simulink model "Stand_Balance"  (R2021b)
settings: Solver=FixedStepDiscrete  StartTime=0.0  StopTime=inf  FixedStep=0.0005  RelTol=1e-3
libraries: simulink x4, IFR_StackLiteDualDrive_SimulinkLib x4
settings Model: Creator=ysl  LastModifiedBy=ysl
settings OptimizationCC: DefaultParameterBehavior=Inlined  EnhancedBackFolding=on  PassReuseOutputArgsAs=Individual arguments  ZeroExternalMemoryAtStartup=off  ZeroInternalMemoryAtStartup=off  OptimizeBlockOrder=speed  DifferentSizesBufferReuse=on  OptimizationCustomize=off  EfficientTunableParamExpr=on
settings DebuggingCC: ParameterTunabilityLossMsg=error
settings SFSimCC: MATLABDynamicMemAlloc=off
settings RTWCC: Description=IFR StackLite-DualDrive Base on stm32f405RGT6  SystemTargetFile=stacklite_dualdrive.tlc  TemplateMakefile=stacklite_dualdrive.tmf  GenerateReport=on
settings CodeAppCC: ForceParamTrailComments=on  IgnoreCustomStorageClasses=off  OperatorAnnotations=on  SimulinkDataObjDesc=on  SFDataObjDesc=on  InsertBlockDesc=on
settings STFCustomTargetCC: TargetLangStandard=C99 (ISO)  MultiwordLength=256  ParMdlRefBuildCompliant=on  CompOptLevelCompliant=on  CombineOutputUpdateFcns=on  ERTCustomFileBanners=on  SupportContinuousTime=off  SupportNonInlinedSFcns=off  RemoveResetFunc=on  MATLABClassNameForMDSCustomization=Simulink.SoftwareTarget.ERTCustomization  CPPClassGenCompliant=on  GRTInterface=off  SystemTargetFile=stacklite_dualdrive.tlc
settings ERTTargetCC: TargetLangStandard=C99 (ISO)  ConcurrentExecutionCompliant=off  ModelStepFunctionPrototypeControlCompliant=off  UseToolchainInfoCompliant=off  InlinedParameterPlacement=NonHierarchical  ERTCustomFileTemplate=example_file_process.tlc

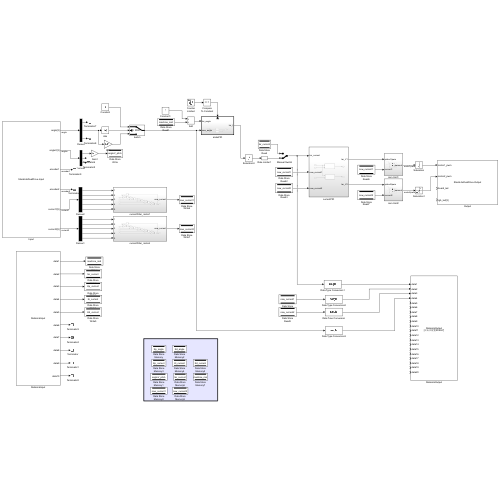
[thumbnail: Simulink's stored preview of the top-level diagram]
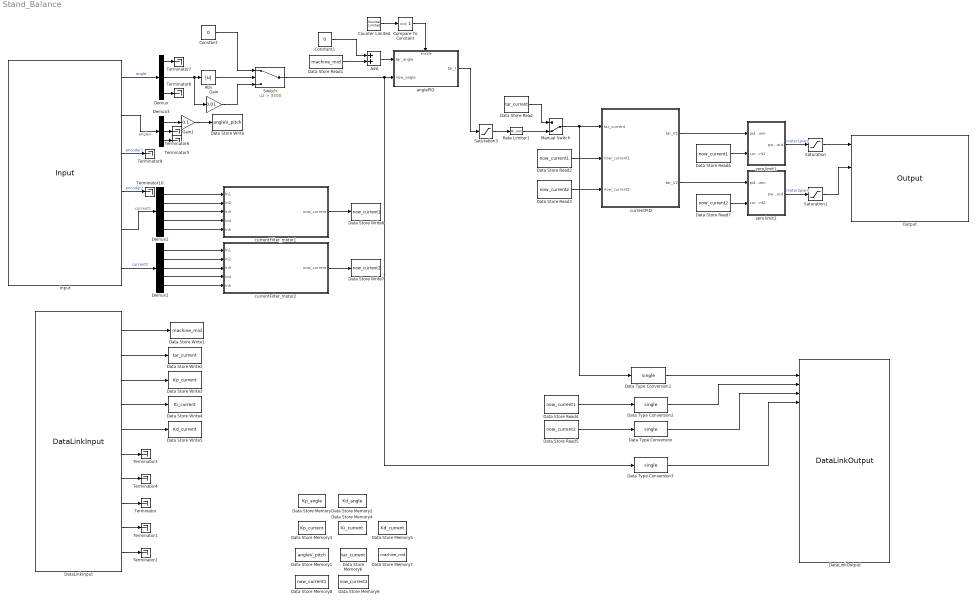
== system Stand_Balance ==
  Abs : Abs
  Add : Sum
  Compare To Constant : simulink/Logic and Bit Operations/Compare To Constant  relop===  const=1  OutDataTypeStr=boolean
  Constant : Constant  Value=0
  Constant1 : Constant  Value=0
  Counter Limited : simulink/Sources/Counter Limited  uplimit=1  tsamp=-1
  Data Store Memory : DataStoreMemory  DataStoreName=Kp_angle  ReadBeforeWriteMsg=warning  WriteAfterWriteMsg=warning  WriteAfterReadMsg=warning  ShowAdditionalParam=off
  Data Store Memory1 : DataStoreMemory  DataStoreName=angleV_pitch  ReadBeforeWriteMsg=warning  WriteAfterWriteMsg=warning  WriteAfterReadMsg=warning  ShowAdditionalParam=off
  Data Store Memory2 : DataStoreMemory  DataStoreName=Kd_angle  ReadBeforeWriteMsg=warning  WriteAfterWriteMsg=warning  WriteAfterReadMsg=warning  ShowAdditionalParam=off
  Data Store Memory3 : DataStoreMemory  DataStoreName=Kp_current  ReadBeforeWriteMsg=warning  WriteAfterWriteMsg=warning  WriteAfterReadMsg=warning  ShowAdditionalParam=off
  Data Store Memory4 : DataStoreMemory  DataStoreName=Ki_current  ReadBeforeWriteMsg=warning  WriteAfterWriteMsg=warning  WriteAfterReadMsg=warning  ShowAdditionalParam=off
  Data Store Memory5 : DataStoreMemory  DataStoreName=Kd_current  ReadBeforeWriteMsg=warning  WriteAfterWriteMsg=warning  WriteAfterReadMsg=warning  ShowAdditionalParam=off
  Data Store Memory6 : DataStoreMemory  DataStoreName=tar_current  ReadBeforeWriteMsg=warning  WriteAfterWriteMsg=warning  WriteAfterReadMsg=warning  ShowAdditionalParam=off
  Data Store Memory7 : DataStoreMemory  DataStoreName=machine_mid  ReadBeforeWriteMsg=warning  WriteAfterWriteMsg=warning  WriteAfterReadMsg=warning  ShowAdditionalParam=off
  Data Store Memory8 : DataStoreMemory  DataStoreName=now_current1  ReadBeforeWriteMsg=warning  WriteAfterWriteMsg=warning  WriteAfterReadMsg=warning  ShowAdditionalParam=off
  Data Store Memory9 : DataStoreMemory  DataStoreName=now_current2  ReadBeforeWriteMsg=warning  WriteAfterWriteMsg=warning  WriteAfterReadMsg=warning  ShowAdditionalParam=off
  Data Store Read : DataStoreRead  DataStoreName=tar_current  IndexOptions=Index vector (dialog)  Indices=1  OutputSizes=1
  Data Store Read1 : DataStoreRead  DataStoreName=machine_mid  IndexOptions=Index vector (dialog)  Indices=1  OutputSizes=1
  Data Store Read2 : DataStoreRead  DataStoreName=now_current1  IndexOptions=Index vector (dialog)  Indices=1  OutputSizes=1
  Data Store Read3 : DataStoreRead  DataStoreName=now_current2  IndexOptions=Index vector (dialog)  Indices=1  OutputSizes=1
  Data Store Read4 : DataStoreRead  DataStoreName=now_current1  IndexOptions=Index vector (dialog)  Indices=1  OutputSizes=1
  Data Store Read5 : DataStoreRead  DataStoreName=now_current2  IndexOptions=Index vector (dialog)  Indices=1  OutputSizes=1
  Data Store Read6 : DataStoreRead  DataStoreName=now_current1  IndexOptions=Index vector (dialog)  Indices=1  OutputSizes=1
  Data Store Read7 : DataStoreRead  DataStoreName=now_current2  IndexOptions=Index vector (dialog)  Indices=1  OutputSizes=1
  Data Store Write : DataStoreWrite  DataStoreName=angleV_pitch  IndexOptions=Index vector (dialog)  Indices=1  OutputSizes=1
  Data Store Write1 : DataStoreWrite  DataStoreName=machine_mid  IndexOptions=Index vector (dialog)  Indices=1  OutputSizes=1
  Data Store Write2 : DataStoreWrite  DataStoreName=tar_current  IndexOptions=Index vector (dialog)  Indices=1  OutputSizes=1
  Data Store Write3 : DataStoreWrite  DataStoreName=Kp_current  IndexOptions=Index vector (dialog)  Indices=1  OutputSizes=1
  Data Store Write4 : DataStoreWrite  DataStoreName=Ki_current  IndexOptions=Index vector (dialog)  Indices=1  OutputSizes=1
  Data Store Write5 : DataStoreWrite  DataStoreName=Kd_current  IndexOptions=Index vector (dialog)  Indices=1  OutputSizes=1
  Data Store Write6 : DataStoreWrite  DataStoreName=now_current1  IndexOptions=Index vector (dialog)  Indices=1  OutputSizes=1
  Data Store Write7 : DataStoreWrite  DataStoreName=now_current2  IndexOptions=Index vector (dialog)  Indices=1  OutputSizes=1
  Data Type Conversion{,1..3} (4 alike) : DataTypeConversion  OutDataTypeStr=single
  DataLinkInput : IFR_StackLiteDualDrive_SimulinkLib/DataLinkInput
      settings: SourceProductName=IFR_StackLiteDualDrive_SimulinkLib_V1.0
  DataLinkOutput : IFR_StackLiteDualDrive_SimulinkLib/DataLinkOutput  id='BalanceUnname'  key='IFR00'
      settings: SourceProductName=IFR_StackLiteDualDrive_SimulinkLib_V1.0
  Demux : Demux  Outputs=3
  Demux1 : Demux  Outputs=5
  Demux2 : Demux  Outputs=5
  Demux3 : Demux  Outputs=3
  Gain : Gain  Gain=0.01
  Gain1 : Gain  Gain=0.1
  Input : IFR_StackLiteDualDrive_SimulinkLib/Input  Priority=0
      settings: SourceProductName=IFR_StackLiteDualDrive_SimulinkLib_V1.0
  Manual Switch : ManualSwitch  CurrentSetting=0
  Output : IFR_StackLiteDualDrive_SimulinkLib/Output  Priority=255
      settings: SourceProductName=IFR_StackLiteDualDrive_SimulinkLib_V1.0
  Rate Limiter1 : RateLimiter  RisingSlewLimit=10000  FallingSlewLimit=-10000  SampleTimeMode=inherited
  Saturation : Saturate  UpperLimit=4200  LowerLimit=-4200
  Saturation1 : Saturate  UpperLimit=4200  LowerLimit=-4200
  Saturation3 : Saturate  UpperLimit=2048  LowerLimit=-2048  OutDataTypeStr=int16
  Switch : Switch  Criteria=u2 > Threshold  Threshold=3500
  Terminator{,1..10} (11 alike) : Terminator
  anglePID : Subsystem
  currentFilter_motor1 : Subsystem
  currentFilter_motor2 : Subsystem
  currentPID : Subsystem
  zero limit1 : Subsystem
  zero limit2 : Subsystem
  wires:
  Input/1 -> Demux/1  "angle"
  Abs/1 -> Switch/2
  Constant/1 -> Switch/1
  Saturation3/1 -> Rate Limiter1/1
  currentPID/1(tar_V1) -> zero limit1/1(pidout1pwm)
  Counter Limited/1 -> Compare To Constant/1
  Compare To Constant/1 -> anglePID/Enable
  Switch/1 -> anglePID/2(now_angle), Data Type Conversion3/1
  anglePID/1(tar_I) -> Saturation3/1
  Constant1/1 -> Add/1
  Data Store Read1/1 -> Add/2
  Add/1 -> anglePID/1(tar_angle)
  Input/6 -> Demux1/1  "current2"
  Input/5 -> Demux2/1  "current1"
  Demux2/1 -> currentFilter_motor1/1(In1)
  Demux2/2 -> currentFilter_motor1/2(In2)
  Demux2/3 -> currentFilter_motor1/3(In3)
  Demux2/5 -> currentFilter_motor1/5(In5)
  Demux1/1 -> currentFilter_motor2/1(In1)
  Demux2/4 -> currentFilter_motor1/4(In4)
  Demux1/2 -> currentFilter_motor2/2(In2)
  Demux1/3 -> currentFilter_motor2/3(In3)
  Demux1/4 -> currentFilter_motor2/4(In4)
  Demux1/5 -> currentFilter_motor2/5(In5)
  currentPID/2(tar_V2) -> zero limit2/1(pidout2pwm)
  zero limit1/1(pwmout) -> Saturation/1  "motor1pwm"
  zero limit2/1(pwmout) -> Saturation1/1  "motor2pwm"
  Saturation1/1 -> Output/2
  Saturation/1 -> Output/1
  Input/2 -> Demux3/1  "anglev"
  Data Store Read/1 -> Manual Switch/1
  Rate Limiter1/1 -> Manual Switch/2
  Manual Switch/1 -> Data Type Conversion1/1, currentPID/1(tar_current)
  DataLinkInput/1 -> Data Store Write1/1
  DataLinkInput/2 -> Data Store Write2/1
  DataLinkInput/3 -> Data Store Write3/1
  DataLinkInput/4 -> Data Store Write4/1
  DataLinkInput/5 -> Data Store Write5/1
  Data Type Conversion1/1 -> DataLinkOutput/1
  Data Type Conversion2/1 -> DataLinkOutput/2
  Data Type Conversion/1 -> DataLinkOutput/3
  Data Type Conversion3/1 -> DataLinkOutput/4
  DataLinkInput/8 -> Terminator/1
  DataLinkInput/9 -> Terminator1/1
  DataLinkInput/10 -> Terminator2/1
  Demux3/3 -> Terminator5/1
  Demux/3 -> Terminator8/1
  Gain1/1 -> Data Store Write/1
  Demux/1 -> Terminator7/1
  Demux/2 -> Gain/1, Abs/1
  Demux3/2 -> Terminator6/1
  Demux3/1 -> Gain1/1
  Gain/1 -> Switch/3
  DataLinkInput/6 -> Terminator3/1
  DataLinkInput/7 -> Terminator4/1
  Input/3 -> Terminator9/1  "encoder1"
  Input/4 -> Terminator10/1  "encoder2"
  currentFilter_motor1/1(now_current) -> Data Store Write6/1
  currentFilter_motor2/1(now_current) -> Data Store Write7/1
  Data Store Read2/1 -> currentPID/2(now_current1)
  Data Store Read3/1 -> currentPID/3(now_current2)
  Data Store Read4/1 -> Data Type Conversion2/1
  Data Store Read5/1 -> Data Type Conversion/1
  Data Store Read6/1 -> zero limit1/2(current1)
  Data Store Read7/1 -> zero limit2/2(current2)

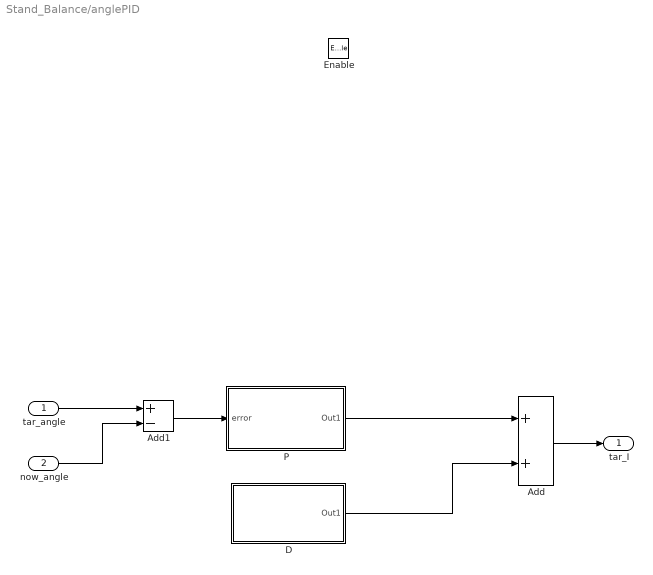
== system Stand_Balance/anglePID ==
  tar_angle : Inport
  now_angle : Inport  Port=2
  Enable : EnablePort
  Add : Sum  OutDataTypeStr=double
  Add1 : Sum  Inputs=+-
  D : Subsystem
  P : Subsystem
  tar_I : Outport
  wires:
  Add/1 -> tar_I/1
  D/1(Out1) -> Add/2
  now_angle/1 -> Add1/2
  tar_angle/1 -> Add1/1
  P/1(Out1) -> Add/1
  Add1/1 -> P/1(error)

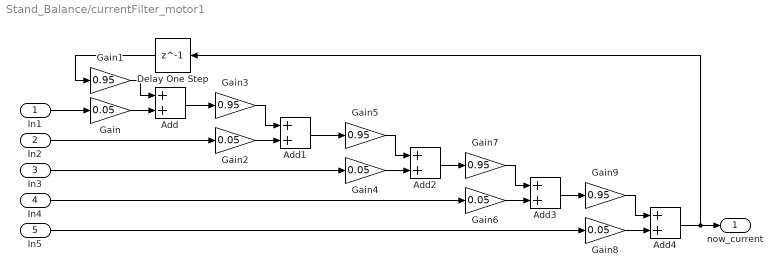
== system Stand_Balance/currentFilter_motor1 ==
  In1 : Inport
  In2 : Inport  Port=2
  In3 : Inport  Port=3
  In4 : Inport  Port=4
  In5 : Inport  Port=5
  Add{,1..4} (5 alike) : Sum
  Delay One Step : Delay  DelayLength=1
  Gain{,2,4,6,8} (5 alike) : Gain  Gain=0.05  OutDataTypeStr=single
  Gain{1,3,5,7,9} (5 alike) : Gain  Gain=0.95  OutDataTypeStr=single
  now_current : Outport
  wires:
  Gain1/1 -> Add/1
  Gain5/1 -> Add2/1
  Gain/1 -> Add/2
  Gain3/1 -> Add1/1
  In2/1 -> Gain2/1
  Gain2/1 -> Add1/2
  Delay One Step/1 -> Gain1/1
  In1/1 -> Gain/1
  Add/1 -> Gain3/1
  Gain4/1 -> Add2/2
  In4/1 -> Gain6/1
  Add1/1 -> Gain5/1
  Gain9/1 -> Add4/1
  Add2/1 -> Gain7/1
  Gain8/1 -> Add4/2
  Gain7/1 -> Add3/1
  Add4/1 -> now_current/1, Delay One Step/1
  Gain6/1 -> Add3/2
  Add3/1 -> Gain9/1
  In5/1 -> Gain8/1
  In3/1 -> Gain4/1

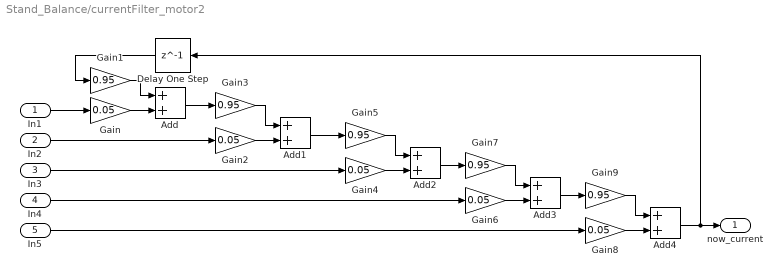
== system Stand_Balance/currentFilter_motor2 ==
  In1 : Inport
  In2 : Inport  Port=2
  In3 : Inport  Port=3
  In4 : Inport  Port=4
  In5 : Inport  Port=5
  Add{,1..4} (5 alike) : Sum
  Delay One Step : Delay  DelayLength=1
  Gain{,2,4,6,8} (5 alike) : Gain  Gain=0.05  OutDataTypeStr=single
  Gain{1,3,5,7,9} (5 alike) : Gain  Gain=0.95  OutDataTypeStr=single
  now_current : Outport
  wires:
  In3/1 -> Gain4/1
  In5/1 -> Gain8/1
  Add3/1 -> Gain9/1
  Gain6/1 -> Add3/2
  Add4/1 -> Delay One Step/1, now_current/1
  Gain7/1 -> Add3/1
  Gain8/1 -> Add4/2
  Add2/1 -> Gain7/1
  Gain9/1 -> Add4/1
  Add1/1 -> Gain5/1
  In4/1 -> Gain6/1
  Gain4/1 -> Add2/2
  Add/1 -> Gain3/1
  In1/1 -> Gain/1
  Delay One Step/1 -> Gain1/1
  Gain2/1 -> Add1/2
  In2/1 -> Gain2/1
  Gain3/1 -> Add1/1
  Gain/1 -> Add/2
  Gain5/1 -> Add2/1
  Gain1/1 -> Add/1

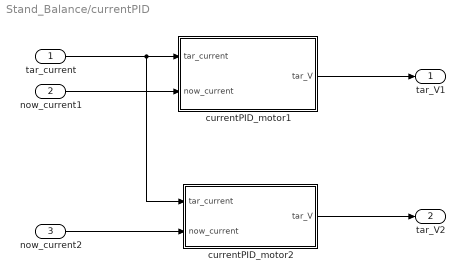
== system Stand_Balance/currentPID ==
  tar_current : Inport
  now_current1 : Inport  Port=2
  now_current2 : Inport  Port=3
  currentPID_motor1 : Subsystem
  currentPID_motor2 : Subsystem
  tar_V1 : Outport
  tar_V2 : Outport  Port=2
  wires:
  tar_current/1 -> currentPID_motor2/1(tar_current), currentPID_motor1/1(tar_current)
  now_current1/1 -> currentPID_motor1/2(now_current)
  currentPID_motor1/1(tar_V) -> tar_V1/1
  now_current2/1 -> currentPID_motor2/2(now_current)
  currentPID_motor2/1(tar_V) -> tar_V2/1

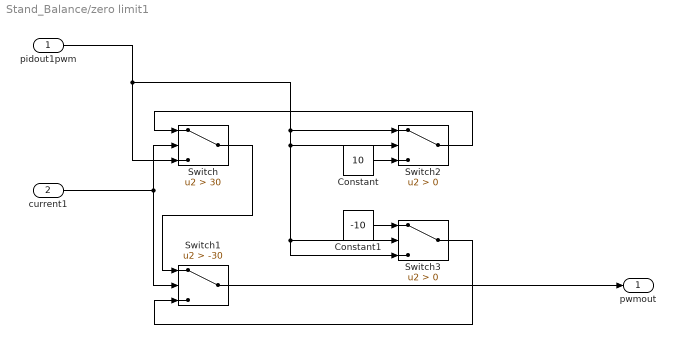
== system Stand_Balance/zero limit1 ==
  pidout1pwm : Inport
  current1 : Inport  Port=2
  Constant : Constant  Value=10  OutDataTypeStr=int16
  Constant1 : Constant  Value=-10  OutDataTypeStr=int16
  Switch : Switch  Criteria=u2 > Threshold  Threshold=30  OutDataTypeStr=int16
  Switch1 : Switch  Criteria=u2 > Threshold  Threshold=-30  OutDataTypeStr=int16
  Switch2 : Switch  Criteria=u2 > Threshold  OutDataTypeStr=int16
  Switch3 : Switch  Criteria=u2 > Threshold  OutDataTypeStr=int16
  pwmout : Outport
  wires:
  Switch1/1 -> pwmout/1
  Switch2/1 -> Switch/1
  Switch3/1 -> Switch1/3
  Switch/1 -> Switch1/1
  Constant/1 -> Switch2/3
  pidout1pwm/1 -> Switch2/2, Switch3/2, Switch3/3, Switch2/1, Switch/3
  current1/1 -> Switch1/2, Switch/2
  Constant1/1 -> Switch3/1

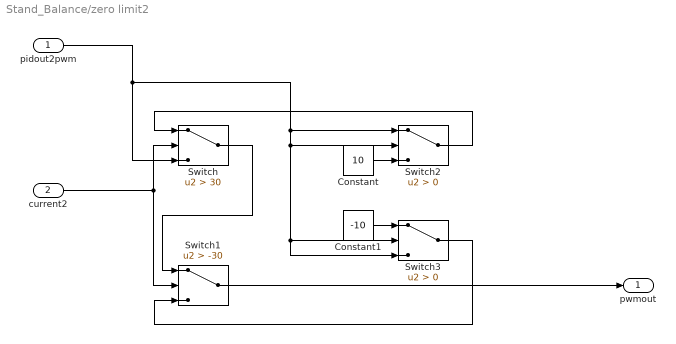
== system Stand_Balance/zero limit2 ==
  pidout2pwm : Inport
  current2 : Inport  Port=2
  Constant : Constant  Value=10  OutDataTypeStr=int16
  Constant1 : Constant  Value=-10  OutDataTypeStr=int16
  Switch : Switch  Criteria=u2 > Threshold  Threshold=30  OutDataTypeStr=int16
  Switch1 : Switch  Criteria=u2 > Threshold  Threshold=-30  OutDataTypeStr=int16
  Switch2 : Switch  Criteria=u2 > Threshold  OutDataTypeStr=int16
  Switch3 : Switch  Criteria=u2 > Threshold  OutDataTypeStr=int16
  pwmout : Outport
  wires:
  Constant1/1 -> Switch3/1
  current2/1 -> Switch/2, Switch1/2
  pidout2pwm/1 -> Switch/3, Switch2/1, Switch3/3, Switch3/2, Switch2/2
  Constant/1 -> Switch2/3
  Switch/1 -> Switch1/1
  Switch3/1 -> Switch1/3
  Switch2/1 -> Switch/1
  Switch1/1 -> pwmout/1

== system Stand_Balance/anglePID/D ==
  Constant2 : Constant  Value=0.1
  Data Store Read : DataStoreRead  DataStoreName=angleV_pitch  IndexOptions=Index vector (dialog)  Indices=1  OutputSizes=1
  Data Store Read2 : DataStoreRead  DataStoreName=Kd_angle  IndexOptions=Index vector (dialog)  Indices=1  OutputSizes=1
  Manual Switch2 : ManualSwitch
  Product2 : Product
  Out1 : Outport
  wires:
  Data Store Read/1 -> Product2/2
  Product2/1 -> Out1/1
  Data Store Read2/1 -> Manual Switch2/2
  Manual Switch2/1 -> Product2/1
  Constant2/1 -> Manual Switch2/1

== system Stand_Balance/anglePID/P ==
  error : Inport
  Constant : Constant  Value=70
  Data Store Read : DataStoreRead  DataStoreName=Kp_angle  IndexOptions=Index vector (dialog)  Indices=1  OutputSizes=1
  Manual Switch : ManualSwitch
  Product : Product
  Out1 : Outport
  wires:
  error/1 -> Product/2
  Manual Switch/1 -> Product/1
  Data Store Read/1 -> Manual Switch/2
  Constant/1 -> Manual Switch/1
  Product/1 -> Out1/1

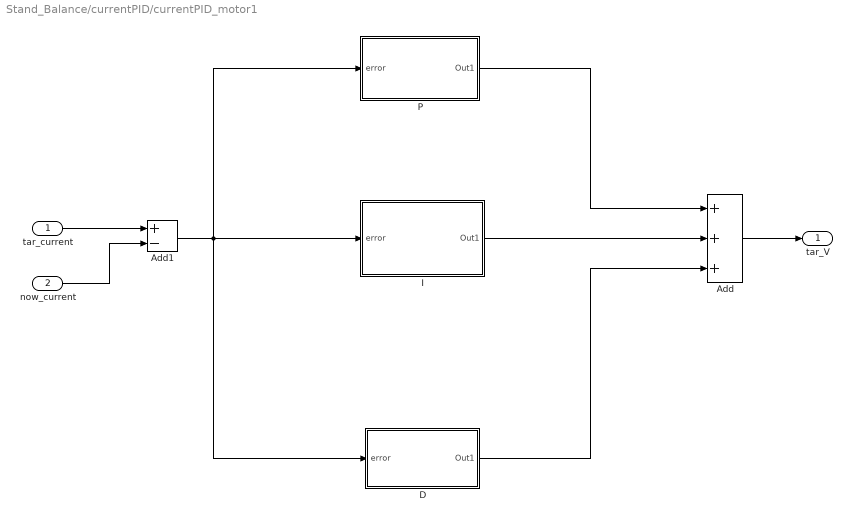
== system Stand_Balance/currentPID/currentPID_motor1 ==
  tar_current : Inport
  now_current : Inport  Port=2
  Add : Sum  Inputs=+++  OutDataTypeStr=double
  Add1 : Sum  Inputs=+-
  D : Subsystem
  I : Subsystem
  P : Subsystem
  tar_V : Outport
  wires:
  I/1(Out1) -> Add/2
  tar_current/1 -> Add1/1
  now_current/1 -> Add1/2
  P/1(Out1) -> Add/1
  Add1/1 -> D/1(error), I/1(error), P/1(error)
  D/1(Out1) -> Add/3
  Add/1 -> tar_V/1

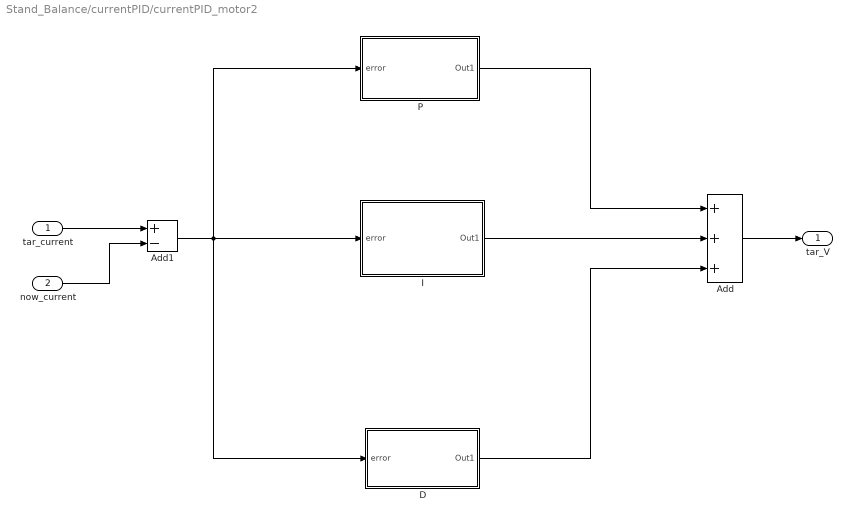
== system Stand_Balance/currentPID/currentPID_motor2 ==
  tar_current : Inport
  now_current : Inport  Port=2
  Add : Sum  Inputs=+++  OutDataTypeStr=double
  Add1 : Sum  Inputs=+-
  D : Subsystem
  I : Subsystem
  P : Subsystem
  tar_V : Outport
  wires:
  Add/1 -> tar_V/1
  D/1(Out1) -> Add/3
  Add1/1 -> P/1(error), I/1(error), D/1(error)
  P/1(Out1) -> Add/1
  now_current/1 -> Add1/2
  tar_current/1 -> Add1/1
  I/1(Out1) -> Add/2

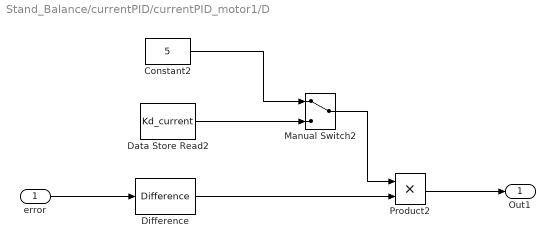
== system Stand_Balance/currentPID/currentPID_motor1/D ==
  error : Inport
  Constant2 : Constant  Value=5
  Data Store Read2 : DataStoreRead  DataStoreName=Kd_current  IndexOptions=Index vector (dialog)  Indices=1  OutputSizes=1
  Difference : simulink/Discrete/Difference  ICPrevInput=0.0  OutMin=[]  OutMax=[]  OutDataType=fixdt(1, 16)  OutScaling=2^-10  DoSatur=off
  Manual Switch2 : ManualSwitch
  Product2 : Product
  Out1 : Outport
  wires:
  Difference/1 -> Product2/2
  Product2/1 -> Out1/1
  Data Store Read2/1 -> Manual Switch2/2
  Manual Switch2/1 -> Product2/1
  Constant2/1 -> Manual Switch2/1
  error/1 -> Difference/1

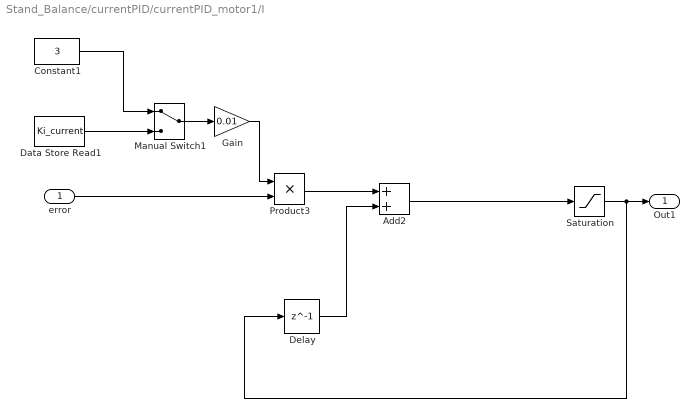
== system Stand_Balance/currentPID/currentPID_motor1/I ==
  error : Inport
  Add2 : Sum
  Constant1 : Constant  Value=3
  Data Store Read1 : DataStoreRead  DataStoreName=Ki_current  IndexOptions=Index vector (dialog)  Indices=1  OutputSizes=1
  Delay : Delay  DelayLength=1
  Gain : Gain  Gain=0.01
  Manual Switch1 : ManualSwitch
  Product3 : Product  OutDataTypeStr=single
  Saturation : Saturate  UpperLimit=2000  LowerLimit=-2000
  Out1 : Outport
  wires:
  Delay/1 -> Add2/2
  Gain/1 -> Product3/1
  Constant1/1 -> Manual Switch1/1
  Manual Switch1/1 -> Gain/1
  Data Store Read1/1 -> Manual Switch1/2
  Product3/1 -> Add2/1
  error/1 -> Product3/2
  Add2/1 -> Saturation/1
  Saturation/1 -> Delay/1, Out1/1

== system Stand_Balance/currentPID/currentPID_motor1/P ==
  error : Inport
  Constant : Constant  Value=7
  Data Store Read : DataStoreRead  DataStoreName=Kp_current  IndexOptions=Index vector (dialog)  Indices=1  OutputSizes=1
  Manual Switch : ManualSwitch
  Product : Product
  Out1 : Outport
  wires:
  error/1 -> Product/2
  Manual Switch/1 -> Product/1
  Data Store Read/1 -> Manual Switch/2
  Constant/1 -> Manual Switch/1
  Product/1 -> Out1/1

== system Stand_Balance/currentPID/currentPID_motor2/D ==
  error : Inport
  Constant2 : Constant  Value=4
  Data Store Read2 : DataStoreRead  DataStoreName=Kd_current  IndexOptions=Index vector (dialog)  Indices=1  OutputSizes=1
  Difference : simulink/Discrete/Difference  ICPrevInput=0.0  OutMin=[]  OutMax=[]  OutDataType=fixdt(1, 16)  OutScaling=2^-10  DoSatur=off
  Manual Switch2 : ManualSwitch
  Product2 : Product
  Out1 : Outport
  wires:
  error/1 -> Difference/1
  Constant2/1 -> Manual Switch2/1
  Manual Switch2/1 -> Product2/1
  Data Store Read2/1 -> Manual Switch2/2
  Product2/1 -> Out1/1
  Difference/1 -> Product2/2

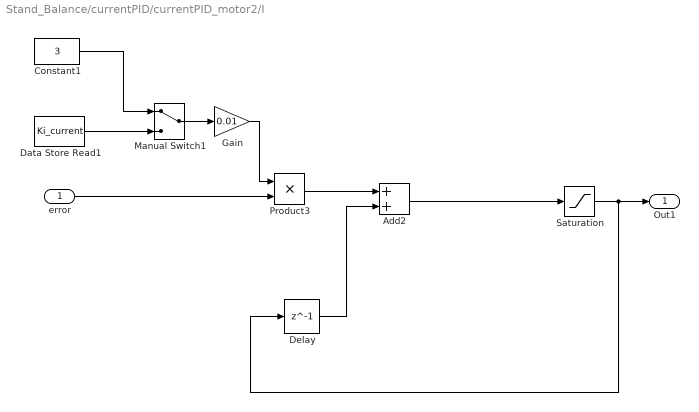
== system Stand_Balance/currentPID/currentPID_motor2/I ==
  error : Inport
  Add2 : Sum
  Constant1 : Constant  Value=3
  Data Store Read1 : DataStoreRead  DataStoreName=Ki_current  IndexOptions=Index vector (dialog)  Indices=1  OutputSizes=1
  Delay : Delay  DelayLength=1
  Gain : Gain  Gain=0.01
  Manual Switch1 : ManualSwitch
  Product3 : Product  OutDataTypeStr=single
  Saturation : Saturate  UpperLimit=2000  LowerLimit=-2000
  Out1 : Outport
  wires:
  Add2/1 -> Saturation/1
  error/1 -> Product3/2
  Product3/1 -> Add2/1
  Data Store Read1/1 -> Manual Switch1/2
  Manual Switch1/1 -> Gain/1
  Constant1/1 -> Manual Switch1/1
  Gain/1 -> Product3/1
  Delay/1 -> Add2/2
  Saturation/1 -> Out1/1, Delay/1

== system Stand_Balance/currentPID/currentPID_motor2/P ==
  error : Inport
  Constant : Constant  Value=7
  Data Store Read : DataStoreRead  DataStoreName=Kp_current  IndexOptions=Index vector (dialog)  Indices=1  OutputSizes=1
  Manual Switch : ManualSwitch
  Product : Product
  Out1 : Outport
  wires:
  Product/1 -> Out1/1
  Constant/1 -> Manual Switch/1
  Data Store Read/1 -> Manual Switch/2
  Manual Switch/1 -> Product/1
  error/1 -> Product/2
